simulink model "hapticForceCtrlr"  (R2025b)
settings: Solver=FixedStepDiscrete  StartTime=0.0  StopTime=inf  FixedStep=0.001  RelTol=1e-3
model workspace (MAT data in the model file):
  p_factor_right = 0.03
  p_gain = 0.03
  udpsocket_id_zone_left = Simulink.Signal
  udpsocket_id_zone_left.Dimensions = 1
  udpsocket_id_zone_left.DimensionsMode = 'auto'
  udpsocket_id_zone_left.Complexity = 'auto'
  udpsocket_id_zone_left.SampleTime = -1
  udpsocket_id_zone_left.SamplingMode = 'auto'
  udpsocket_id_zone_left.InitialValue = '-1'
  udpsocket_id_zone_left.DataType = 'int32'
  udpsocket_id_zone_right = Simulink.Signal
  udpsocket_id_zone_right.Dimensions = 1
  udpsocket_id_zone_right.DimensionsMode = 'auto'
  udpsocket_id_zone_right.Complexity = 'auto'
  udpsocket_id_zone_right.SampleTime = -1
  udpsocket_id_zone_right.SamplingMode = 'auto'
  udpsocket_id_zone_right.InitialValue = '-1'
  udpsocket_id_zone_right.DataType = 'int32'
libraries: simulink x13, simulink_extras x2
settings Model: Creator=KAL82WI  LastModifiedBy=GXC2KOR
settings DataIOCC: DSMLogging=off  SaveTime=off  ReturnWorkspaceOutputs=off
settings OptimizationCC: EnhancedBackFolding=on  PassReuseOutputArgsAs=Individual arguments  ZeroExternalMemoryAtStartup=off  ZeroInternalMemoryAtStartup=off  OptimizeBlockOrder=speed  DifferentSizesBufferReuse=on  EfficientTunableParamExpr=on
settings DebuggingCC: ParameterTunabilityLossMsg=error
settings HardwareCC: ProdBitPerLong=64.0  ProdLargestAtomicInteger=LongLong  ProdLargestAtomicFloat=Double  ProdLongLongMode=on  ProdHWDeviceType=ARM Compatible->ARM Cortex-A (64-bit)
settings SFSimCC: SimUserSources=da_connector.cpp  SimUserIncludeDirs=..\src  MATLABDynamicMemAlloc=off  CustomCodeUndefinedFunction=UseInterfaceOnly  SimTargetLang=C++  SimDLTargetLibrary=mkl-dnn
settings SFSimCC: SimCustomHeaderCode=|
  | serializer.hpp
  | udpcom.hpp
  | da_connector.hpp
settings RTWCC: SystemTargetFile=ert.tlc  HardwareBoard=Example SSH Board  TemplateMakefile=ert_default_tmf  CustomDefine=EXTMODE_SAMPLING_RATE_HZ=100  Toolchain=Remote SSH Build Toolchain  BuildConfiguration=Release  TargetLang=C++  Description=Embedded Coder
settings RTWCC: CustomHeaderCode=|
  | serializer.hpp
  | udpcom.hpp
  | da_connector.hpp
  | types.grpc.pb.h
  | types.pb.h
  | val.grpc.pb.h
  | val.pb.h
settings RTWCC: CustomInclude=|
  | ..\src
  | ..\src\local\protogen
  | ..\src\local\protogen\kuksa\val\v1
  | .\src\rpi_libs
settings RTWCC: CustomSource=|
  | ..\src\serializer.cpp
  | ..\src\udpcom.cpp
  | ..\src\da_connector.cpp
  | ..\src\client.cpp
  | ..\src\local\protogen\kuksa\val\v1\val.pb.cpp
  | ..\src\local\protogen\kuksa\val\v1\val.grpc.pb.cpp
  | ..\src\local\protogen\kuksa\val\v1\types.pb.cpp
  | ..\src\local\protogen\kuksa\val\v1\types.grpc.pb.cpp
settings RTWCC: CustomLibrary=|
  | ..\src\rpi_libs\libgrpc++.so.1.51
  | ..\src\rpi_libs\libprotobuf.so.32
  | ..\src\rpi_libs\libgrpc.so
  | ..\src\rpi_libs\libgpr.so
  | ..\src\rpi_libs\libabsl_synchronization.so.20220623
  | ..\src\rpi_libs\libabsl_time.so.20220623
  | ..\src\rpi_libs\libabsl_strings.so.20220623
  | ..\src\rpi_libs\libabsl_base.so.20220623
  | ..\src\rpi_libs\libpthread.so.0
  | ..\src\rpi_libs\libdl.so.2
  | ..\src\rpi_libs\libstdc++.so.6
  | ..\src\rpi_libs\libm.so.6
  | ..\src\rpi_libs\librt.so.1
settings CodeAppCC: ForceParamTrailComments=on  IgnoreCustomStorageClasses=off  OperatorAnnotations=on  SimulinkDataObjDesc=on  SFDataObjDesc=on  InsertBlockDesc=on
settings ERTTargetCC: ExtMode=on  ExtModeStaticAlloc=on  ExtModeMexFile=ext_xcp  ExtModeIntrfLevel=Level2 - Open  InlinedParameterPlacement=Hierarchical  ERTCustomFileTemplate=example_file_process.tlc  TargetLangStandard=C++11 (ISO)  GenerateSampleERTMain=on  SupportNonInlinedSFcns=on

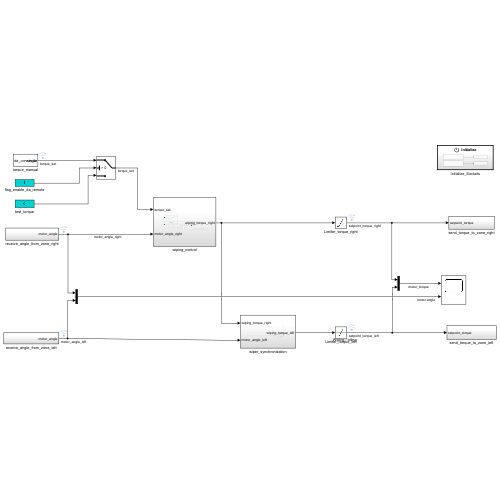
[thumbnail: Simulink's stored preview of the top-level diagram]
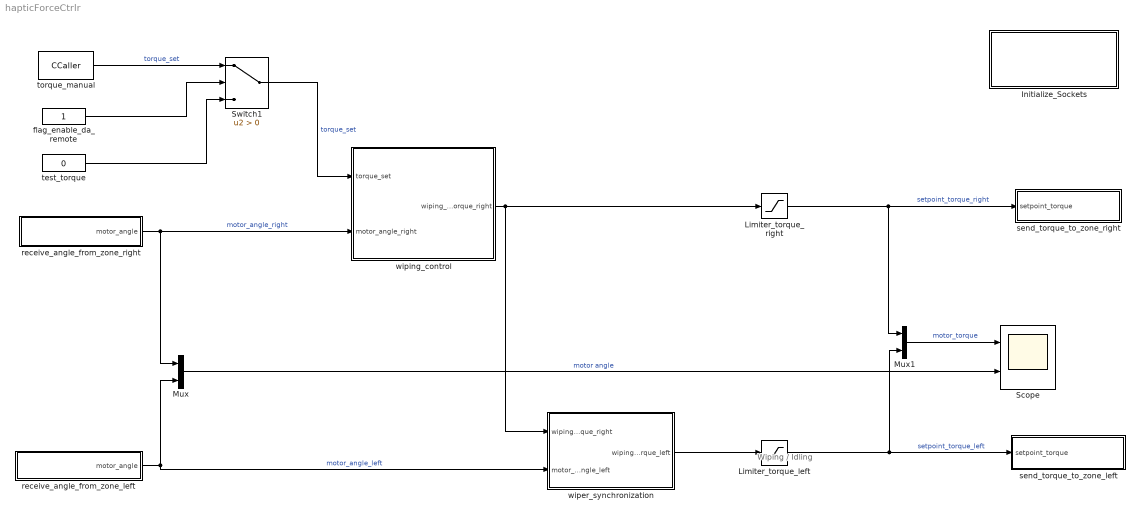
== system hapticForceCtrlr ==
  note: Wiping / Idling
  Initialize_Sockets : Subsystem  TreatAsAtomicUnit=on
  Limiter_torque_left : Saturate  UpperLimit=10  LowerLimit=-10
  Limiter_torque_right : Saturate  UpperLimit=10  LowerLimit=-10
  Mux : Mux  Inputs=2
  Mux1 : Mux  Inputs=2
  Scope : Scope  NumInputPorts=2
      settings: ActiveDisplayYMinimum=-43.454094564953081  ActiveDisplayYMaximum=10.429521695951717
  Switch1 : Switch  Criteria=u2 > Threshold  SaturateOnIntegerOverflow=off  InputSameDT=off
  flag_enable_da_remote : Constant  OutDataTypeStr=boolean
  receive_angle_from_zone_left : Subsystem
  receive_angle_from_zone_right : Subsystem
  send_torque_to_zone_left : Subsystem
  send_torque_to_zone_right : Subsystem
  test_torque : Constant  Value=0  OutMin=-1000.0  OutMax=10000.0  OutDataTypeStr=single
  torque_manual : CCaller  FunctionName=da_connector  PortSpecificationStruct="%)30     .    ( (   8    (     @         %    \"     $    !     0         %  0 \"0    $    _    07)G3F%M90  4&]R=$YA;64 4V-O<&4     26YD97@     5'EP90      4VEZ90      27-';&]B86P   X    P    !@    @    $          4    (     0    ,    !         !   P!O=70 #@   #@    &    \"     0         !0    @    !    !@    $         $     8   !S:6YG;&4   X    X    !@    @    $          4    (     0    8    !         !     &    3W5T<'5T   .    .     8    (    !@         %    \"     $    !     0         )    \"               #@   #@    &    \"     0         !0    @    !    !@    $         $     8   !D;W5B;&4   X    P    !@    @    $          4    (     0    $    !         !   0 Q    #@   #     &    \"     D\"        !0    @    !     0    $          @ !"
  wiper_synchronization : Subsystem
  wiping_control : Subsystem
  wires:
  wiping_control/1(wiping_torque_right) -> Limiter_torque_right/1, wiper_synchronization/1(wiping_torque_right)
  Limiter_torque_right/1 -> Mux1/1, send_torque_to_zone_right/1(setpoint_torque)  "setpoint_torque_right"
  receive_angle_from_zone_right/1(motor_angle) -> Mux/1, wiping_control/2(motor_angle_right)  "motor_angle_right"
  receive_angle_from_zone_left/1(motor_angle) -> Mux/2, wiper_synchronization/2(motor_angle_left)  "motor_angle_left"
  Limiter_torque_left/1 -> Mux1/2, send_torque_to_zone_left/1(setpoint_torque)  "setpoint_torque_left"
  Switch1/1 -> wiping_control/1(torque_set)  "torque_set"
  torque_manual/1 -> Switch1/1  "torque_set"
  flag_enable_da_remote/1 -> Switch1/2
  test_torque/1 -> Switch1/3
  wiper_synchronization/1(wiping_torque_left) -> Limiter_torque_left/1
  Mux/1 -> Scope/2  "motor angle"
  Mux1/1 -> Scope/1  "motor_torque"

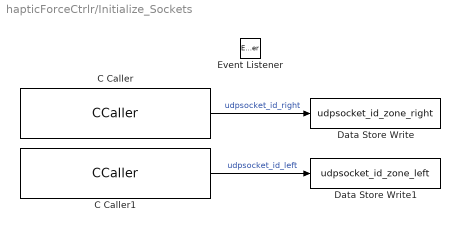
== system hapticForceCtrlr/Initialize_Sockets ==
  C Caller : CCaller  FunctionName=ini_udp_socket  PortSpecificationStruct="%)30     .    * (   8    (     @         %    \"     $    !     0         %  0 \"0    $    _    07)G3F%M90  4&]R=$YA;64 4V-O<&4     26YD97@     5'EP90      4VEZ90      27-';&]B86P   X    P    !@    @    $          4    (     0    ,    !         !   P!O=70 #@   $     &    \"     0         !0    @    !    \"0    $         $     D   !U9'!S;V-K970         #@   #@    &    \"     0         !0    @    !    !@    $         $     8   !/=71P=70   X    X    !@    @    &          4    (     0    $    !          D    (               .    .     8    (    !          %    \"     $    %     0         0    !0   &EN=#,R    #@   #     &    \"     0         !0    @    !     0    $         $  ! #$    .    ,     8    (    \"0(        %    \"     $    !     0         \"  $"
  C Caller1 : CCaller  FunctionName=ini_udp_socket  PortSpecificationStruct="%)30     .    * (   8    (     @         %    \"     $    !     0         %  0 \"0    $    _    07)G3F%M90  4&]R=$YA;64 4V-O<&4     26YD97@     5'EP90      4VEZ90      27-';&]B86P   X    P    !@    @    $          4    (     0    ,    !         !   P!O=70 #@   $     &    \"     0         !0    @    !    \"0    $         $     D   !U9'!S;V-K970         #@   #@    &    \"     0         !0    @    !    !@    $         $     8   !/=71P=70   X    X    !@    @    &          4    (     0    $    !          D    (               .    .     8    (    !          %    \"     $    %     0         0    !0   &EN=#,R    #@   #     &    \"     0         !0    @    !     0    $         $  ! #$    .    ,     8    (    \"0(        %    \"     $    !     0         \"  $"
  Data Store Write : DataStoreWrite  DataStoreName=udpsocket_id_zone_right  DataStoreElements=udpsocket_id_zone_right  IndexOptions=Index vector (dialog)  Indices=1  OutputSizes=1
  Data Store Write1 : DataStoreWrite  DataStoreName=udpsocket_id_zone_left  DataStoreElements=udpsocket_id_zone_left  IndexOptions=Index vector (dialog)  Indices=1  OutputSizes=1
  Event Listener : EventListener  DisableCoverage=on  EventName=reset
  wires:
  C Caller/1 -> Data Store Write/1  "udpsocket_id_right"
  C Caller1/1 -> Data Store Write1/1  "udpsocket_id_left"

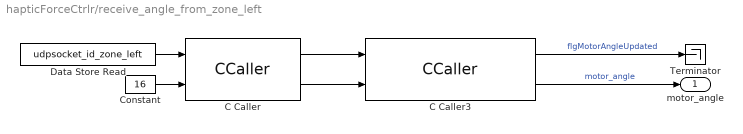
== system hapticForceCtrlr/receive_angle_from_zone_left ==
  C Caller : CCaller  FunctionName=udpreceive  PortSpecificationStruct="%)30     .    0 <   8    (     @         %    \"     0    !     0         %  0 \"0    $    _    07)G3F%M90  4&]R=$YA;64 4V-O<&4     26YD97@     5'EP90      4VEZ90      27-';&]B86P   X    P    !@    @    $          4    (     0    ,    !         !   P!O=70 #@   #@    &    \"     0         !0    @    !    \"     $         $     @   !L96Y?9&%T80X    X    !@    @    $          4    (     0    8    !   ...(+2119 chars)"
  C Caller3 : CCaller  FunctionName=deserializeFields  PortSpecificationStruct="%)30     .    8 <   8    (     @         %    \"     0    !     0         %  0 \"0    $    _    07)G3F%M90  4&]R=$YA;64 4V-O<&4     26YD97@     5'EP90      4VEZ90      27-';&]B86P   X    P    !@    @    $          4    (     0    ,    !         !   P!O=70 #@   $@    &    \"     0         !0    @    !    %     $         $    !0   !F;&=-;W1O<D%N9VQE57!D871E9      .    .     8    (    !          %    ...(+2163 chars)"
  Constant : Constant  Value=16  OutDataTypeStr=Inherit: Inherit via back propagation
  Data Store Read : DataStoreRead  DataStoreName=udpsocket_id_zone_left  DataStoreElements=udpsocket_id_zone_left  IndexOptions=Index vector (dialog)  Indices=1  OutputSizes=1
  Terminator : Terminator
  motor_angle : Outport
  wires:
  C Caller/1 -> C Caller3/1
  C Caller/2 -> C Caller3/2
  C Caller3/2 -> motor_angle/1  "motor_angle"
  Constant/1 -> C Caller/2
  Data Store Read/1 -> C Caller/1
  C Caller3/1 -> Terminator/1  "flgMotorAngleUpdated"

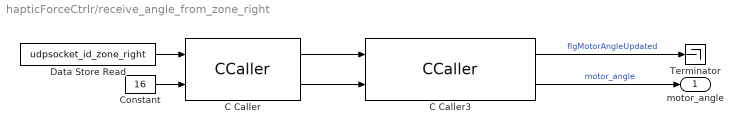
== system hapticForceCtrlr/receive_angle_from_zone_right ==
  C Caller : CCaller  FunctionName=udpreceive  PortSpecificationStruct="%)30     .    0 <   8    (     @         %    \"     0    !     0         %  0 \"0    $    _    07)G3F%M90  4&]R=$YA;64 4V-O<&4     26YD97@     5'EP90      4VEZ90      27-';&]B86P   X    P    !@    @    $          4    (     0    ,    !         !   P!O=70 #@   #@    &    \"     0         !0    @    !    \"     $         $     @   !L96Y?9&%T80X    X    !@    @    $          4    (     0    8    !   ...(+2119 chars)"
  C Caller3 : CCaller  FunctionName=deserializeFields  PortSpecificationStruct="%)30     .    8 <   8    (     @         %    \"     0    !     0         %  0 \"0    $    _    07)G3F%M90  4&]R=$YA;64 4V-O<&4     26YD97@     5'EP90      4VEZ90      27-';&]B86P   X    P    !@    @    $          4    (     0    ,    !         !   P!O=70 #@   $@    &    \"     0         !0    @    !    %     $         $    !0   !F;&=-;W1O<D%N9VQE57!D871E9      .    .     8    (    !          %    ...(+2163 chars)"
  Constant : Constant  Value=16  OutDataTypeStr=Inherit: Inherit via back propagation
  Data Store Read : DataStoreRead  DataStoreName=udpsocket_id_zone_right  DataStoreElements=udpsocket_id_zone_right  IndexOptions=Index vector (dialog)  Indices=1  OutputSizes=1
  Terminator : Terminator
  motor_angle : Outport
  wires:
  C Caller/1 -> C Caller3/1
  C Caller/2 -> C Caller3/2
  C Caller3/2 -> motor_angle/1  "motor_angle"
  Constant/1 -> C Caller/2
  Data Store Read/1 -> C Caller/1
  C Caller3/1 -> Terminator/1  "flgMotorAngleUpdated"

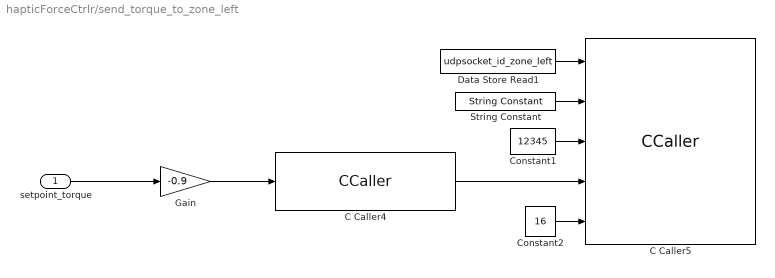
== system hapticForceCtrlr/send_torque_to_zone_left ==
  setpoint_torque : Inport
  C Caller4 : CCaller  FunctionName=serializeFields  PortSpecificationStruct="%)30     .    Z ,   8    (     @         %    \"     (    !     0         %  0 \"0    $    _    07)G3F%M90  4&]R=$YA;64 4V-O<&4     26YD97@     5'EP90      4VEZ90      27-';&]B86P   X   !     !@    @    $          4    (     0    H    !         !     *    <V5T7W1O<G%U90        X   !     !@    @    $          4    (     0    H    !         !     *    <V5T7W1O<G%U90        X    X    !@    @    $          4    (     0    4    !         !     %    26YP=70    .    .     8    (    !@         %    \"     $    !     0         )    \"               #@   #@    &    \"     0         !0    @    !    !@    $         $     8   !S:6YG;&4   X    P    !@    @    $          4    (     0    $    !         !   0 Q    #@   #     &    \"     D\"        !0    @    !     0    $          @ !       .    .     8    (    !          %    \"     $    &     0         0    !@   &)U9F9E<@  #@   #@    &    \"     0         !0    @    !    !@    $         $     8   !B=69F97(   X    X    !@    @    $          4    (     0    8    !         !     &    3W5T<'5T   .    .     8    (    !@         %    \"     $    !     0         )    \"               #@   #@    &    \"     0         !0    @    !    !0    $         $     4   !U:6YT.     X    P    !@    @    $          4    (     0    (    !         !   @ Q-@  #@   #     &    \"     D\"        !0    @    !     0    $          @ !"
  C Caller5 : CCaller  FunctionName=udpsend  PortSpecificationStruct="%)30     .    & D   8    (     @         %    \"     4    !     0         %  0 \"0    $    _    07)G3F%M90  4&]R=$YA;64 4V-O<&4     26YD97@     5'EP90      4VEZ90      27-';&]B86P   X    X    !@    @    $          4    (     0    8    !         !     &    <V]C:V9D   .    .     8    (    !          %    \"     $    &     0         0    !@   '-O8VMF9   #@   #@    &    \"     0         !0    @    !   ...(+2755 chars)"
  Constant1 : Constant  Value=12345  OutDataTypeStr=uint16
  Constant2 : Constant  Value=16  OutDataTypeStr=Inherit: Inherit via back propagation
  Data Store Read1 : DataStoreRead  DataStoreName=udpsocket_id_zone_left  DataStoreElements=udpsocket_id_zone_left  IndexOptions=Index vector (dialog)  Indices=1  OutputSizes=1
  Gain : Gain  Gain=-0.9  OutDataTypeStr=single
  String Constant : StringConstant  String="\"192.168.88.21\""
  wires:
  Constant1/1 -> C Caller5/3
  C Caller4/1 -> C Caller5/4
  Constant2/1 -> C Caller5/5
  Data Store Read1/1 -> C Caller5/1
  String Constant/1 -> C Caller5/2
  setpoint_torque/1 -> Gain/1
  Gain/1 -> C Caller4/1

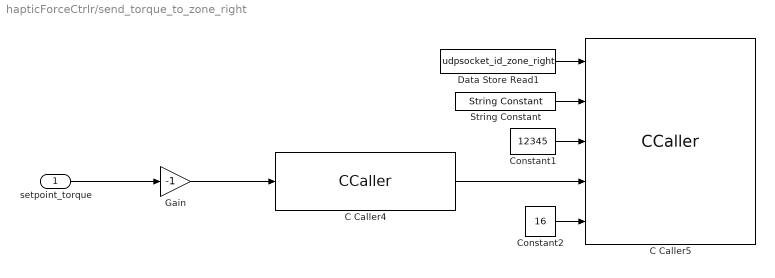
== system hapticForceCtrlr/send_torque_to_zone_right ==
  setpoint_torque : Inport
  C Caller4 : CCaller  FunctionName=serializeFields  PortSpecificationStruct="%)30     .    Z ,   8    (     @         %    \"     (    !     0         %  0 \"0    $    _    07)G3F%M90  4&]R=$YA;64 4V-O<&4     26YD97@     5'EP90      4VEZ90      27-';&]B86P   X   !     !@    @    $          4    (     0    H    !         !     *    <V5T7W1O<G%U90        X   !     !@    @    $          4    (     0    H    !         !     *    <V5T7W1O<G%U90        X    X    !@    @    $          4    (     0    4    !         !     %    26YP=70    .    .     8    (    !@         %    \"     $    !     0         )    \"               #@   #@    &    \"     0         !0    @    !    !@    $         $     8   !S:6YG;&4   X    P    !@    @    $          4    (     0    $    !         !   0 Q    #@   #     &    \"     D\"        !0    @    !     0    $          @ !       .    .     8    (    !          %    \"     $    &     0         0    !@   &)U9F9E<@  #@   #@    &    \"     0         !0    @    !    !@    $         $     8   !B=69F97(   X    X    !@    @    $          4    (     0    8    !         !     &    3W5T<'5T   .    .     8    (    !@         %    \"     $    !     0         )    \"               #@   #@    &    \"     0         !0    @    !    !0    $         $     4   !U:6YT.     X    P    !@    @    $          4    (     0    (    !         !   @ Q-@  #@   #     &    \"     D\"        !0    @    !     0    $          @ !"
  C Caller5 : CCaller  FunctionName=udpsend  PortSpecificationStruct="%)30     .    & D   8    (     @         %    \"     4    !     0         %  0 \"0    $    _    07)G3F%M90  4&]R=$YA;64 4V-O<&4     26YD97@     5'EP90      4VEZ90      27-';&]B86P   X    X    !@    @    $          4    (     0    8    !         !     &    <V]C:V9D   .    .     8    (    !          %    \"     $    &     0         0    !@   '-O8VMF9   #@   #@    &    \"     0         !0    @    !   ...(+2755 chars)"
  Constant1 : Constant  Value=12345  OutDataTypeStr=uint16
  Constant2 : Constant  Value=16  OutDataTypeStr=Inherit: Inherit via back propagation
  Data Store Read1 : DataStoreRead  DataStoreName=udpsocket_id_zone_right  DataStoreElements=udpsocket_id_zone_right  IndexOptions=Index vector (dialog)  Indices=1  OutputSizes=1
  Gain : Gain  Gain=-1  OutDataTypeStr=single
  String Constant : StringConstant  String="\"192.168.88.22\""
  wires:
  Constant1/1 -> C Caller5/3
  C Caller4/1 -> C Caller5/4
  Constant2/1 -> C Caller5/5
  Data Store Read1/1 -> C Caller5/1
  String Constant/1 -> C Caller5/2
  setpoint_torque/1 -> Gain/1
  Gain/1 -> C Caller4/1

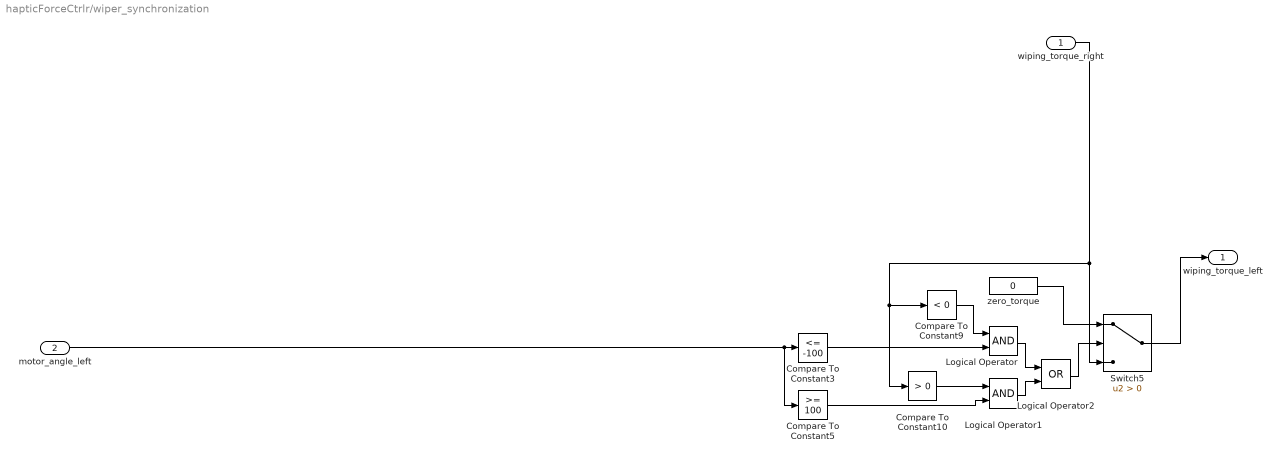
== system hapticForceCtrlr/wiper_synchronization ==
  wiping_torque_right : Inport
  motor_angle_left : Inport  Port=2
  Compare To Constant10 : simulink/Logic and Bit Operations/Compare To Constant  relop=>  const=0  OutDataTypeStr=boolean
  Compare To Constant3 : simulink/Logic and Bit Operations/Compare To Constant  relop=<=  const=-100  OutDataTypeStr=boolean
  Compare To Constant5 : simulink/Logic and Bit Operations/Compare To Constant  relop=>=  const=100  OutDataTypeStr=boolean
  Compare To Constant9 : simulink/Logic and Bit Operations/Compare To Constant  relop=<  const=0  OutDataTypeStr=boolean
  Logical Operator : Logic  AllPortsSameDT=off  OutDataTypeStr=boolean
  Logical Operator1 : Logic  AllPortsSameDT=off  OutDataTypeStr=boolean
  Logical Operator2 : Logic  Operator=OR  AllPortsSameDT=off  OutDataTypeStr=boolean
  Switch5 : Switch  Criteria=u2 > Threshold  OutDataTypeStr=single  SaturateOnIntegerOverflow=off  InputSameDT=off
  zero_torque : Constant  Value=0  OutDataTypeStr=boolean
  wiping_torque_left : Outport
  wires:
  Logical Operator2/1 -> Switch5/2
  motor_angle_left/1 -> Compare To Constant5/1, Compare To Constant3/1
  wiping_torque_right/1 -> Compare To Constant10/1, Compare To Constant9/1, Switch5/3
  Compare To Constant9/1 -> Logical Operator/1
  Compare To Constant10/1 -> Logical Operator1/1
  Compare To Constant5/1 -> Logical Operator1/2
  Compare To Constant3/1 -> Logical Operator/2
  Logical Operator/1 -> Logical Operator2/1
  Logical Operator1/1 -> Logical Operator2/2
  Switch5/1 -> wiping_torque_left/1
  zero_torque/1 -> Switch5/1

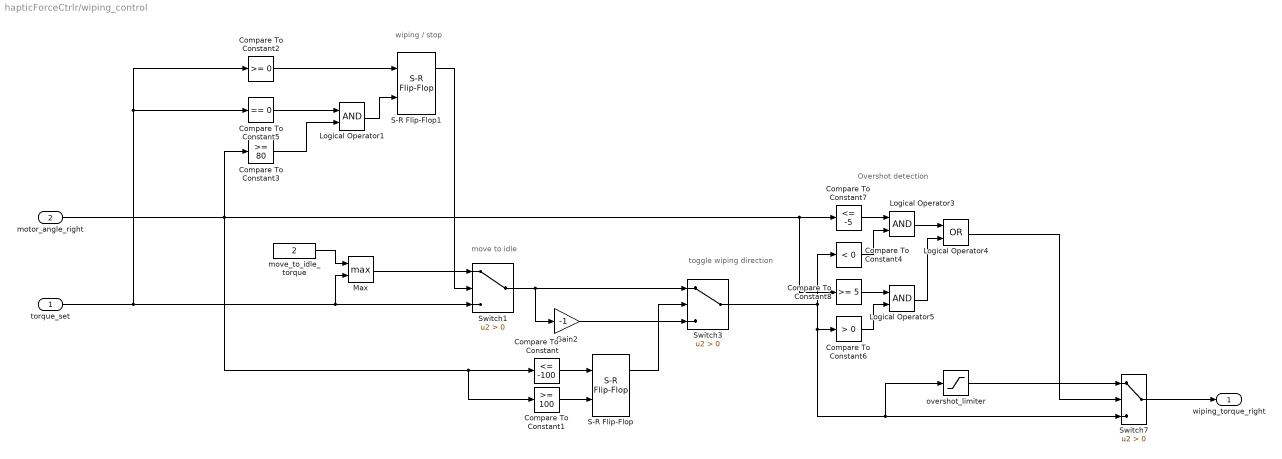
== system hapticForceCtrlr/wiping_control ==
  note: Overshot detection
  note: toggle wiping direction
  note: move to idle
  note: wiping / stop
  torque_set : Inport
  motor_angle_right : Inport  Port=2
  Compare To Constant : simulink/Logic and Bit Operations/Compare To Constant  relop=<=  const=-100  OutDataTypeStr=boolean
  Compare To Constant1 : simulink/Logic and Bit Operations/Compare To Constant  relop=>=  const=100  OutDataTypeStr=boolean
  Compare To Constant2 : simulink/Logic and Bit Operations/Compare To Constant  relop=>=  const=0  OutDataTypeStr=boolean
  Compare To Constant3 : simulink/Logic and Bit Operations/Compare To Constant  relop=>=  const=80  OutDataTypeStr=boolean
  Compare To Constant4 : simulink/Logic and Bit Operations/Compare To Constant  relop=<  const=0  OutDataTypeStr=boolean
  Compare To Constant5 : simulink/Logic and Bit Operations/Compare To Constant  relop===  const=0  OutDataTypeStr=boolean
  Compare To Constant6 : simulink/Logic and Bit Operations/Compare To Constant  relop=>  const=0  OutDataTypeStr=boolean
  Compare To Constant7 : simulink/Logic and Bit Operations/Compare To Constant  relop=<=  const=-5  OutDataTypeStr=boolean
  Compare To Constant8 : simulink/Logic and Bit Operations/Compare To Constant  relop=>=  const=5  OutDataTypeStr=boolean
  Gain2 : Gain  Gain=-1
  Logical Operator1 : Logic  AllPortsSameDT=off  OutDataTypeStr=boolean
  Logical Operator3 : Logic  AllPortsSameDT=off  OutDataTypeStr=boolean
  Logical Operator4 : Logic  Operator=OR  AllPortsSameDT=off  OutDataTypeStr=boolean
  Logical Operator5 : Logic  AllPortsSameDT=off  OutDataTypeStr=boolean
  Max : MinMax  Function=max  Inputs=2
  S-R Flip-Flop : simulink_extras/Flip Flops/S-R Flip-Flop  initial_condition=0
  S-R Flip-Flop1 : simulink_extras/Flip Flops/S-R Flip-Flop  initial_condition=0
  Switch1 : Switch  Criteria=u2 > Threshold  OutDataTypeStr=single  SaturateOnIntegerOverflow=off  InputSameDT=off
  Switch3 : Switch  Criteria=u2 > Threshold  OutDataTypeStr=single  SaturateOnIntegerOverflow=off  InputSameDT=off
  Switch7 : Switch  Criteria=u2 > Threshold  OutDataTypeStr=single  SaturateOnIntegerOverflow=off  InputSameDT=off
  move_to_idle_torque : Constant  Value=2  OutDataTypeStr=double
  overshot_limiter : Saturate  UpperLimit=2  LowerLimit=-2
  wiping_torque_right : Outport
  wires:
  Gain2/1 -> Switch3/3
  overshot_limiter/1 -> Switch7/1
  Switch3/1 -> Compare To Constant6/1, Switch7/3, overshot_limiter/1, Compare To Constant4/1
  motor_angle_right/1 -> Compare To Constant7/1, Compare To Constant8/1, Compare To Constant/1, Compare To Constant1/1, Compare To Constant3/1
  Compare To Constant6/1 -> Logical Operator5/2
  Compare To Constant/1 -> S-R Flip-Flop/1
  Logical Operator5/1 -> Logical Operator4/2
  Compare To Constant1/1 -> S-R Flip-Flop/2
  Compare To Constant8/1 -> Logical Operator5/1
  torque_set/1 -> Max/2, Switch1/3, Compare To Constant2/1, Compare To Constant5/1
  S-R Flip-Flop/1 -> Switch3/2
  Logical Operator3/1 -> Logical Operator4/1
  Compare To Constant4/1 -> Logical Operator3/2
  Compare To Constant7/1 -> Logical Operator3/1
  Logical Operator4/1 -> Switch7/2
  Switch7/1 -> wiping_torque_right/1
  Compare To Constant2/1 -> S-R Flip-Flop1/1
  Logical Operator1/1 -> S-R Flip-Flop1/2
  Switch1/1 -> Switch3/1, Gain2/1
  Max/1 -> Switch1/1
  S-R Flip-Flop1/1 -> Switch1/2
  move_to_idle_torque/1 -> Max/1
  Compare To Constant5/1 -> Logical Operator1/1
  Compare To Constant3/1 -> Logical Operator1/2
